simulink model "testboard_UW_GNCDE"  (R2019a)
settings: Solver=FixedStepAuto  StartTime=0.0  StopTime=100  FixedStep=0.05  RelTol=1e-3
values from neighbouring files (symbols this model uses):
  D = zeros(6,3)    [MPCController_test.m]
undefined symbols (not defined in the file or in its folder): Continuous, DiscIntNeverNeededParam, MPCController_test, MPCController_testq, Time
libraries: aerolibutil x23, sharedtransform x5, simulink_extras x4, simulink x4, sharedutil x4, ephemeris x3, sb_quatrans x3, ATV_cowell_plus_tides x2, FO_frame_q x2, FO_ang_vel x2, reference_frame_inv_change x2, sb_qua2con x2
(part 3 of 3)

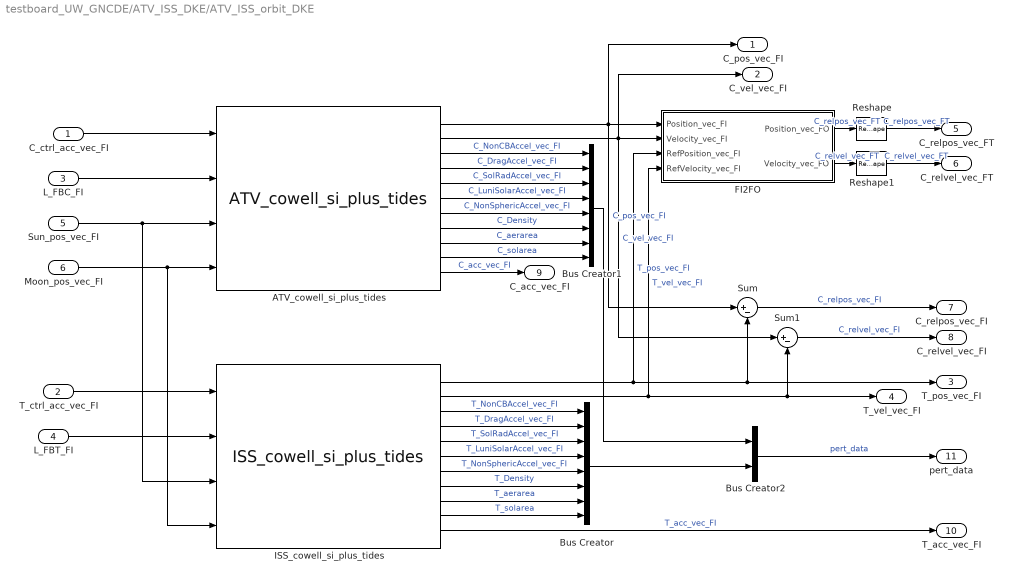
== system testboard_UW_GNCDE/ATV_ISS_DKE/ATV_ISS_orbit_DKE ==
  C_ctrl_acc_vec_FI : Inport
  T_ctrl_acc_vec_FI : Inport  Port=2
  L_FBC_FI : Inport  Port=3
  L_FBT_FI : Inport  Port=4
  Sun_pos_vec_FI : Inport  Port=5
  Moon_pos_vec_FI : Inport  Port=6
  ATV_cowell_si_plus_tides : ATV_cowell_plus_tides/ATV_cowell_si_plus_tides  DiagCtrlNo=6  Ini_option=Specify via Dialog  InitFileName=RVDLEO_test_ATV_cowell_si_plus_tides_init.m  NewFile_Action=Cancel  OldFile_Action=Cancel  InitStatus=on  Ini_Epoch=5479  SC=struct('Ini_Position_vec_FI',[6828447.574;-6.2113;-7.8374],'Ini_Velocity_vec_FI',[3.9161017425529252;4745.7279805152566;5987.6184957602281],'Mass',10,'Cd',2.5,'ReflecCoef',1.3,'stype',3,'aeroa0',0,'solara0',0,'aerob',0,'solarb',0,'XCBdim',0.03,'YCBdim',0.02,'ZCBdim',0.06,'XSAdim',0.03,'YSAdim',0,'ZSAdim',0.06,'SAOrientation',-3,'AeroDragSurface',21,'SolRadSurface',40,'RES_MAG_DIR',1.0000000000000001e-05,'RES_MAG',[1 1 1],'C_COM_FGC',[0 0 0])  AeroDrag_flag=1  SolRad_flag=1  LuniSolar_flag=1  NonSpheric_flag=1  NumZonalTerms=8  NumTessTerms=2  Constants=struct('EarthRadius',6378137,'EarthMu',398600448073446,'SunMu',132712438000000010000,'MoonMu',4902799063000,'SolRadConstant',99060619577789600,'EarthDipoleLong',2.9426251188624395,'EarthDipoleCoelev',1.9120081955597878,'EarthDipole',7943000000000000)
  Bus Creator : BusCreator  Inputs=8
  Bus Creator1 : BusCreator  Inputs=8
  Bus Creator2 : BusCreator  Inputs=2
  FI2FO : Subsystem  AncestorBlock=FI_2_FO/FI2FO
  ISS_cowell_si_plus_tides : ISS_cowell_plus_tides/ISS_cowell_si_plus_tides  DiagCtrlNo=6  Ini_option=Specify via Dialog  InitFileName=RVDLEO_test_ISS_cowell_si_plus_tides_init.m  NewFile_Action=Cancel  OldFile_Action=Cancel  InitStatus=on  Ini_Epoch=5479  SC=struct('Ini_Position_vec_FI',[6828447.574;0;0],'Ini_Velocity_vec_FI',[0;4745.7279805152566;5987.6184957602281],'Mass',10,'Cd',2.5,'ReflecCoef',1.3,'stype',3,'aeroa0',0,'solara0',0,'aerob',0,'solarb',0,'XCBdim',0.03,'YCBdim',0.02,'ZCBdim',0.06,'XSAdim',0.03,'YSAdim',0,'ZSAdim',0.06,'SAOrientation',-3,'AeroDragSurface',0.02,'SolRadSurface',0.06)  AeroDrag_flag=1  SolRad_flag=1  LuniSolar_flag=1  NonSpheric_flag=1  NumZonalTerms=8  NumTessTerms=2  Constants=struct('EarthRadius',6378137,'EarthMu',398600448073446,'SunMu',132712438000000010000,'MoonMu',4902799063000,'SolRadConstant',99060619577789600,'EarthDipoleLong',2.9426251188624395,'EarthDipoleCoelev',1.9120081955597878,'EarthDipole',7943000000000000)
  Reshape : Reshape
  Reshape1 : Reshape
  Sum : Sum  Inputs=|+-  SaturateOnIntegerOverflow=on  InputSameDT=on  OutDataTypeStr=Inherit: Same as first input
  Sum1 : Sum  Inputs=|+-  SaturateOnIntegerOverflow=on  InputSameDT=on  OutDataTypeStr=Inherit: Same as first input
  C_pos_vec_FI : Outport
  C_vel_vec_FI : Outport  Port=2
  T_pos_vec_FI : Outport  Port=3
  T_vel_vec_FI : Outport  Port=4
  C_relpos_vec_FT : Outport  Port=5
  C_relvel_vec_FT : Outport  Port=6
  C_relpos_vec_FI : Outport  Port=7
  C_relvel_vec_FI : Outport  Port=8
  C_acc_vec_FI : Outport  Port=9
  T_acc_vec_FI : Outport  Port=10
  pert_data : Outport  Port=11
  wires:
  Bus Creator/1 -> Bus Creator2/2
  Bus Creator1/1 -> Bus Creator2/1
  ISS_cowell_si_plus_tides/10 -> Bus Creator/8  "T_solarea"
  ISS_cowell_si_plus_tides/9 -> Bus Creator/7  "T_aerarea"
  ISS_cowell_si_plus_tides/8 -> Bus Creator/6  "T_Density"
  ISS_cowell_si_plus_tides/7 -> Bus Creator/5  "T_NonSphericAccel_vec_FI"
  ISS_cowell_si_plus_tides/6 -> Bus Creator/4  "T_LuniSolarAccel_vec_FI"
  ISS_cowell_si_plus_tides/5 -> Bus Creator/3  "T_SolRadAccel_vec_FI"
  ISS_cowell_si_plus_tides/4 -> Bus Creator/2  "T_DragAccel_vec_FI"
  ISS_cowell_si_plus_tides/3 -> Bus Creator/1  "T_NonCBAccel_vec_FI"
  L_FBT_FI/1 -> ISS_cowell_si_plus_tides/2
  T_ctrl_acc_vec_FI/1 -> ISS_cowell_si_plus_tides/1
  Moon_pos_vec_FI/1 -> ATV_cowell_si_plus_tides/4, ISS_cowell_si_plus_tides/4
  Sun_pos_vec_FI/1 -> ATV_cowell_si_plus_tides/3, ISS_cowell_si_plus_tides/3
  L_FBC_FI/1 -> ATV_cowell_si_plus_tides/2
  C_ctrl_acc_vec_FI/1 -> ATV_cowell_si_plus_tides/1
  ATV_cowell_si_plus_tides/10 -> Bus Creator1/8  "C_solarea"
  ATV_cowell_si_plus_tides/8 -> Bus Creator1/6  "C_Density"
  ATV_cowell_si_plus_tides/7 -> Bus Creator1/5  "C_NonSphericAccel_vec_FI"
  ATV_cowell_si_plus_tides/6 -> Bus Creator1/4  "C_LuniSolarAccel_vec_FI"
  ATV_cowell_si_plus_tides/5 -> Bus Creator1/3  "C_SolRadAccel_vec_FI"
  ATV_cowell_si_plus_tides/4 -> Bus Creator1/2  "C_DragAccel_vec_FI"
  ATV_cowell_si_plus_tides/3 -> Bus Creator1/1  "C_NonCBAccel_vec_FI"
  ISS_cowell_si_plus_tides/11 -> T_acc_vec_FI/1  "T_acc_vec_FI"
  ATV_cowell_si_plus_tides/11 -> C_acc_vec_FI/1  "C_acc_vec_FI"
  Bus Creator2/1 -> pert_data/1  "pert_data"
  Sum1/1 -> C_relvel_vec_FI/1  "C_relvel_vec_FI"
  Sum/1 -> C_relpos_vec_FI/1  "C_relpos_vec_FI"
  Reshape1/1 -> C_relvel_vec_FT/1  "C_relvel_vec_FT"
  Reshape/1 -> C_relpos_vec_FT/1  "C_relpos_vec_FT"
  ISS_cowell_si_plus_tides/2 -> T_vel_vec_FI/1, Sum1/2, FI2FO/4(RefVelocity_vec_FI)  "T_vel_vec_FI"
  ISS_cowell_si_plus_tides/1 -> Sum/2, T_pos_vec_FI/1, FI2FO/3(RefPosition_vec_FI)  "T_pos_vec_FI"
  ATV_cowell_si_plus_tides/2 -> C_vel_vec_FI/1, Sum1/1, FI2FO/2(Velocity_vec_FI)  "C_vel_vec_FI"
  ATV_cowell_si_plus_tides/1 -> Sum/1, FI2FO/1(Position_vec_FI), C_pos_vec_FI/1  "C_pos_vec_FI"
  ATV_cowell_si_plus_tides/9 -> Bus Creator1/7  "C_aerarea"
  FI2FO/1(Position_vec_FO) -> Reshape/1  "C_relpos_vec_FT"
  FI2FO/2(Velocity_vec_FO) -> Reshape1/1  "C_relvel_vec_FT"

== system testboard_UW_GNCDE/Dynamic Prototype/Chaser attitude1 ==
  Torque : Inport
  Integrator : Integrator  InitialCondition="[0.2685   -0.1449    0.1277  0.9437]"
  Integrator2 : Integrator  InitialCondition=[2 2 2]*pi/180
  Mux : Mux  Inputs=3
  Mux1 : Mux  Inputs=2
  Td : Constant  Value=ones(3,1)*1e-4
  qdot : MATLABFcn  MATLABFcn=qdot  OutputDimensions=4
  qnorm : MATLAB Function  Commented=on  TreatAsAtomicUnit=on
  wdot1 : MATLABFcn  MATLABFcn=wdot_c  OutputDimensions=3
  q_chaser : Outport
  w_chaser : Outport  Port=2
  wires:
  Integrator2/1 -> Mux1/2, Mux/1, w_chaser/1
  Torque/1 -> Mux/3
  wdot1/1 -> Integrator2/1
  Mux/1 -> wdot1/1
  qdot/1 -> Integrator/1
  Mux1/1 -> qdot/1
  Integrator/1 -> q_chaser/1, Mux1/1
  Td/1 -> Mux/2

== system testboard_UW_GNCDE/Dynamic Prototype/Subsystem1 ==
  q_c : Inport
  q_t : Inport  Port=2
  Quaternion Inverse : aerolibutil/Quaternion Inverse
      settings: SourceProductName=Aerospace Blockset
  Quaternion Multiplication : aerolibutil/Quaternion Multiplication
  q_error : Outport
  wires:
  q_t/1 -> Quaternion Multiplication/1
  q_c/1 -> Quaternion Inverse/1
  Quaternion Inverse/1 -> Quaternion Multiplication/2
  Quaternion Multiplication/1 -> q_error/1

== system testboard_UW_GNCDE/Dynamic Prototype/Target attitude1 ==
  Integrator : Integrator  InitialCondition=[0 0 0 1]
  Integrator2 : Integrator  InitialCondition=[2 2 2]*pi/180*0.01
  MATLAB Function : MATLAB Function  Commented=on  TreatAsAtomicUnit=on
  Mux1 : Mux  Inputs=2
  qdot : MATLABFcn  MATLABFcn=qdot  OutputDimensions=4
  wdot_t : MATLABFcn  MATLABFcn=wdot_t  OutputDimensions=3
  q_target : Outport
  w_target : Outport  Port=2
  wires:
  wdot_t/1 -> Integrator2/1
  Mux1/1 -> qdot/1
  qdot/1 -> Integrator/1
  Integrator/1 -> q_target/1, Mux1/1
  Integrator2/1 -> wdot_t/1, w_target/1, Mux1/2

== system testboard_UW_GNCDE/RVDsensor/coordinate ==
  q_FI_FC : Inport
  q_FI_FT : Inport  Port=2
  Discrete Derivative : simulink/Discrete/Discrete Derivative  gainval=1  ICPrevScaledInput=0.0  OutMin=[]  OutMax=[]  OutDataType=fixdt(1, 16)  OutScaling=2^-10  DoSatur=off
  MATLAB Function1 : MATLAB Function  TreatAsAtomicUnit=on
  Quaternion Multiplication : aerolibutil/Quaternion Multiplication
  Random Number : RandomNumber  Mean=[0;0;0]  Variance=[0.003;0.003;0.003]*0  Seed=[0;0;0]  SampleTime=0.05
  Rotation Angles to Quaternions : sharedtransform/Rotation Angles to Quaternions  rotationOrder=ZYX  aMode=aMode
      settings: SourceProductName=Aerospace Blockset  SourceProductBaseCode=AE
  Unit Delay : UnitDelay  InitialCondition=[0.9515;0.0381;0.1893;0.2393]  SampleTime=-1  HasFrameUpgradeWarning=on
  q_t2c : Subsystem
  RVD_q_FI_FT : Outport
  RVD_w_FT : Outport  Port=2
  wires:
  q_FI_FT/1 -> q_t2c/2(q_t)
  q_FI_FC/1 -> q_t2c/1(q_c)
  Discrete Derivative/1 -> MATLAB Function1/2(qe)
  MATLAB Function1/1(w) -> RVD_w_FT/1
  q_t2c/1(RVD_q_FI_FT) -> Quaternion Multiplication/1
  Unit Delay/1 -> MATLAB Function1/1(u)
  Random Number/1 -> Rotation Angles to Quaternions/1
  Quaternion Multiplication/1 -> Discrete Derivative/1, Unit Delay/1, RVD_q_FI_FT/1
  Rotation Angles to Quaternions/1 -> Quaternion Multiplication/2

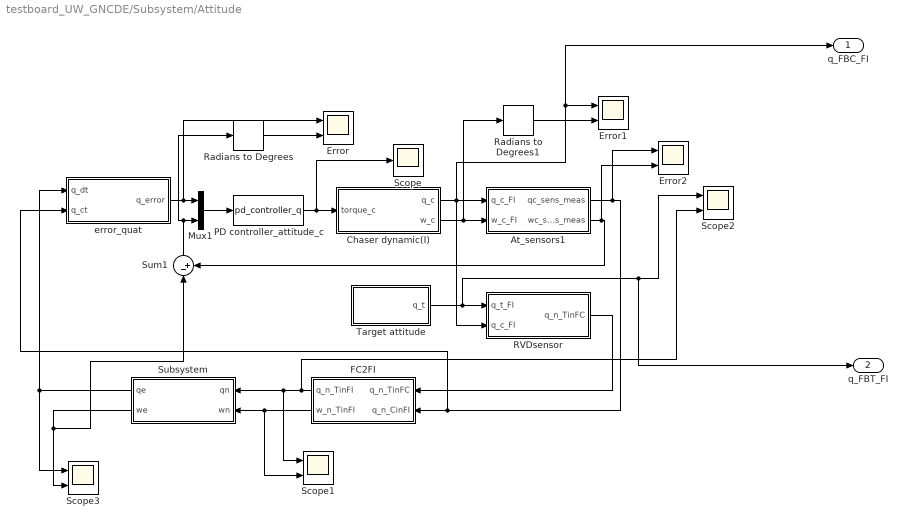
== system testboard_UW_GNCDE/Subsystem/Attitude ==
  At_sensors1 : Subsystem
  Chaser dynamic(I) : Subsystem
  Error : Scope  NumInputPorts=2
  Error1 : Scope  NumInputPorts=2
  Error2 : Scope  NumInputPorts=2
  FC2FI : Subsystem
  Mux1 : Mux  Inputs=2
  PD controller_attitude_c : MATLABFcn  MATLABFcn=pd_controller_q  OutputDimensions=3
  RVDsensor : Subsystem
  Radians to Degrees : simulink_extras/Transformations/Radians to Degrees
  Radians to Degrees1 : simulink_extras/Transformations/Radians to Degrees
  Scope : Scope
  Scope1 : Scope  NumInputPorts=2
  Scope2 : Scope  NumInputPorts=2
  Scope3 : Scope  NumInputPorts=2
  Subsystem : Subsystem
  Sum1 : Sum  Inputs=|-+
  Target attitude : Subsystem
  error_quat : Subsystem
  q_FBC_FI : Outport
  q_FBT_FI : Outport  Port=2
  wires:
  FC2FI/1(q_n_TinFI) -> Scope2/2, Scope1/1, Subsystem/1(qn)
  error_quat/1(q_error) -> Error/1, Mux1/1
  Radians to Degrees1/1 -> Error1/2
  Subsystem/1(qe) -> error_quat/1(q_dt), Scope3/1
  Subsystem/2(we) -> Sum1/1, Scope3/2
  RVDsensor/1(q_n_TinFC) -> FC2FI/1(q_n_TinFC)
  Radians to Degrees/1 -> Error/2
  FC2FI/2(w_n_TinFI) -> Scope1/2, Subsystem/2(wn)
  At_sensors1/2(wc_sens_meas) -> Error2/2, Sum1/2
  Sum1/1 -> Radians to Degrees/1, Mux1/2
  Chaser dynamic(I)/2(w_c) -> Radians to Degrees1/1, At_sensors1/2(w_c_FI)
  Mux1/1 -> PD controller_attitude_c/1
  PD controller_attitude_c/1 -> Scope/1, Chaser dynamic(I)/1(torque_c)
  At_sensors1/1(qc_sens_meas) -> Error2/1, error_quat/2(q_ct), FC2FI/2(q_n_CinFI)
  Chaser dynamic(I)/1(q_c) -> RVDsensor/2(q_c_FI), At_sensors1/1(q_c_FI), q_FBC_FI/1, Error1/1
  Target attitude/1(q_t) -> q_FBT_FI/1, Scope2/1, RVDsensor/1(q_t_FI)

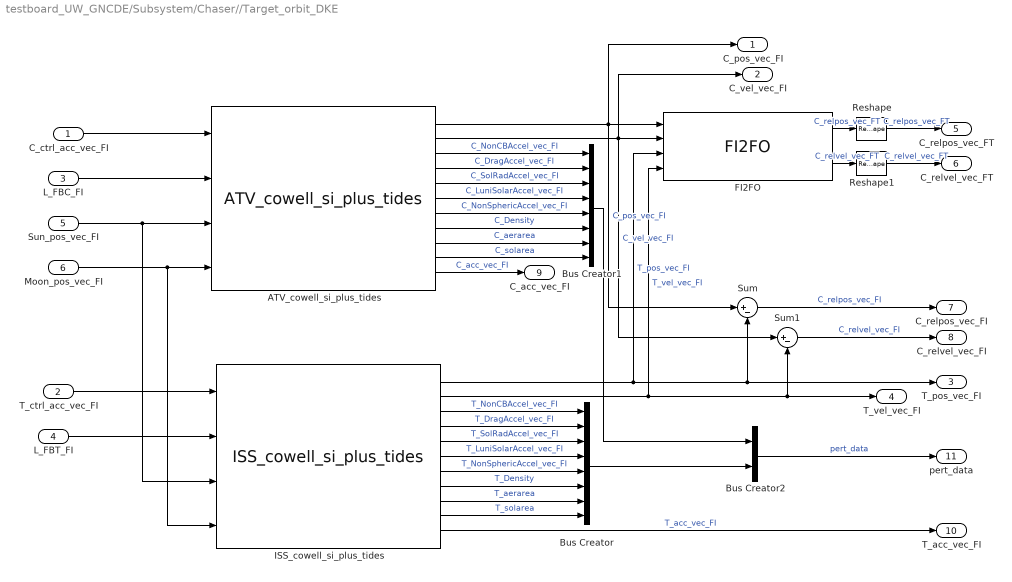
== system testboard_UW_GNCDE/Subsystem/Chaser//Target_orbit_DKE ==
  C_ctrl_acc_vec_FI : Inport
  T_ctrl_acc_vec_FI : Inport  Port=2
  L_FBC_FI : Inport  Port=3
  L_FBT_FI : Inport  Port=4
  Sun_pos_vec_FI : Inport  Port=5
  Moon_pos_vec_FI : Inport  Port=6
  ATV_cowell_si_plus_tides : ATV_cowell_plus_tides/ATV_cowell_si_plus_tides  DiagCtrlNo=6  Ini_option=Specify via Dialog  InitFileName=D:\GNCDE\working_folder\ATV_cowell_si_plus_tides_init.m  NewFile_Action=Cancel  OldFile_Action=Cancel  InitStatus=on  Ini_Epoch=5479  SC=struct('Ini_Position_vec_FI',[6828447.574;-2174.0172420255426;-2742.9270918811635],'Ini_Velocity_vec_FI',[3.9161017425529252;4745.7279805152566;5987.6184957602281],'Mass',10,'Cd',2.5,'ReflecCoef',1.3,'stype',3,'aeroa0',0,'solara0',0,'aerob',0,'solarb',0,'XCBdim',9,'YCBdim',4.5,'ZCBdim',4.5,'XSAdim',0,'YSAdim',5.5,'ZSAdim',5.5,'SAOrientation',-3,'AeroDragSurface',21,'SolRadSurface',40,'RES_MAG_DIR',1.0000000000000001e-05,'RES_MAG',[1 1 1],'C_COM_FGC',[0 0 0])  AeroDrag_flag=1  SolRad_flag=1  LuniSolar_flag=1  NonSpheric_flag=1  NumZonalTerms=8  NumTessTerms=2  Constants=struct('EarthRadius',6378137,'EarthMu',398600448073446,'SunMu',132712438000000010000,'MoonMu',4902799063000,'SolRadConstant',99060619577789600,'EarthDipoleLong',2.9426251188624395,'EarthDipoleCoelev',1.9120081955597878,'EarthDipole',7943000000000000)
  Bus Creator : BusCreator  Inputs=8
  Bus Creator1 : BusCreator  Inputs=8
  Bus Creator2 : BusCreator  Inputs=2
  FI2FO : FI_2_FO/FI2FO  SystemSampleTime=-1
  ISS_cowell_si_plus_tides : ISS_cowell_plus_tides/ISS_cowell_si_plus_tides  DiagCtrlNo=6  Ini_option=Specify via Dialog  InitFileName=D:\GNCDE\working_folder\ISS_cowell_si_plus_tides_init.m  NewFile_Action=Cancel  OldFile_Action=Cancel  InitStatus=on  Ini_Epoch=5479  SC=struct('Ini_Position_vec_FI',[6828447.574;0;0],'Ini_Velocity_vec_FI',[0;4745.7279805152566;5987.6184957602281],'Mass',10,'Cd',2.5,'ReflecCoef',1.3,'stype',3,'aeroa0',0,'solara0',0,'aerob',0,'solarb',0,'XCBdim',54,'YCBdim',65,'ZCBdim',15,'XSAdim',0,'YSAdim',0,'ZSAdim',0,'SAOrientation',-3,'AeroDragSurface',1000,'SolRadSurface',1600)  AeroDrag_flag=1  SolRad_flag=1  LuniSolar_flag=1  NonSpheric_flag=1  NumZonalTerms=8  NumTessTerms=2  Constants=struct('EarthRadius',6378137,'EarthMu',398600448073446,'SunMu',132712438000000010000,'MoonMu',4902799063000,'SolRadConstant',99060619577789600,'EarthDipoleLong',2.9426251188624395,'EarthDipoleCoelev',1.9120081955597878,'EarthDipole',7943000000000000)
  Reshape : Reshape
  Reshape1 : Reshape
  Sum : Sum  Inputs=|+-  SaturateOnIntegerOverflow=on  InputSameDT=on  OutDataTypeStr=Inherit: Same as first input
  Sum1 : Sum  Inputs=|+-  SaturateOnIntegerOverflow=on  InputSameDT=on  OutDataTypeStr=Inherit: Same as first input
  C_pos_vec_FI : Outport
  C_vel_vec_FI : Outport  Port=2
  T_pos_vec_FI : Outport  Port=3
  T_vel_vec_FI : Outport  Port=4
  C_relpos_vec_FT : Outport  Port=5
  C_relvel_vec_FT : Outport  Port=6
  C_relpos_vec_FI : Outport  Port=7
  C_relvel_vec_FI : Outport  Port=8
  C_acc_vec_FI : Outport  Port=9
  T_acc_vec_FI : Outport  Port=10
  pert_data : Outport  Port=11
  wires:
  Bus Creator/1 -> Bus Creator2/2
  Bus Creator1/1 -> Bus Creator2/1
  ISS_cowell_si_plus_tides/10 -> Bus Creator/8  "T_solarea"
  ISS_cowell_si_plus_tides/9 -> Bus Creator/7  "T_aerarea"
  ISS_cowell_si_plus_tides/8 -> Bus Creator/6  "T_Density"
  ISS_cowell_si_plus_tides/7 -> Bus Creator/5  "T_NonSphericAccel_vec_FI"
  ISS_cowell_si_plus_tides/6 -> Bus Creator/4  "T_LuniSolarAccel_vec_FI"
  ISS_cowell_si_plus_tides/5 -> Bus Creator/3  "T_SolRadAccel_vec_FI"
  ISS_cowell_si_plus_tides/4 -> Bus Creator/2  "T_DragAccel_vec_FI"
  ISS_cowell_si_plus_tides/3 -> Bus Creator/1  "T_NonCBAccel_vec_FI"
  L_FBT_FI/1 -> ISS_cowell_si_plus_tides/2
  T_ctrl_acc_vec_FI/1 -> ISS_cowell_si_plus_tides/1
  Moon_pos_vec_FI/1 -> ATV_cowell_si_plus_tides/4, ISS_cowell_si_plus_tides/4
  Sun_pos_vec_FI/1 -> ATV_cowell_si_plus_tides/3, ISS_cowell_si_plus_tides/3
  L_FBC_FI/1 -> ATV_cowell_si_plus_tides/2
  C_ctrl_acc_vec_FI/1 -> ATV_cowell_si_plus_tides/1
  ATV_cowell_si_plus_tides/10 -> Bus Creator1/8  "C_solarea"
  ATV_cowell_si_plus_tides/8 -> Bus Creator1/6  "C_Density"
  ATV_cowell_si_plus_tides/7 -> Bus Creator1/5  "C_NonSphericAccel_vec_FI"
  ATV_cowell_si_plus_tides/6 -> Bus Creator1/4  "C_LuniSolarAccel_vec_FI"
  ATV_cowell_si_plus_tides/5 -> Bus Creator1/3  "C_SolRadAccel_vec_FI"
  ATV_cowell_si_plus_tides/4 -> Bus Creator1/2  "C_DragAccel_vec_FI"
  ATV_cowell_si_plus_tides/3 -> Bus Creator1/1  "C_NonCBAccel_vec_FI"
  ISS_cowell_si_plus_tides/11 -> T_acc_vec_FI/1  "T_acc_vec_FI"
  ATV_cowell_si_plus_tides/11 -> C_acc_vec_FI/1  "C_acc_vec_FI"
  Bus Creator2/1 -> pert_data/1  "pert_data"
  Sum1/1 -> C_relvel_vec_FI/1  "C_relvel_vec_FI"
  Sum/1 -> C_relpos_vec_FI/1  "C_relpos_vec_FI"
  Reshape1/1 -> C_relvel_vec_FT/1  "C_relvel_vec_FT"
  Reshape/1 -> C_relpos_vec_FT/1  "C_relpos_vec_FT"
  ISS_cowell_si_plus_tides/2 -> T_vel_vec_FI/1, Sum1/2, FI2FO/4  "T_vel_vec_FI"
  ISS_cowell_si_plus_tides/1 -> Sum/2, T_pos_vec_FI/1, FI2FO/3  "T_pos_vec_FI"
  ATV_cowell_si_plus_tides/2 -> C_vel_vec_FI/1, Sum1/1, FI2FO/2  "C_vel_vec_FI"
  ATV_cowell_si_plus_tides/1 -> Sum/1, FI2FO/1, C_pos_vec_FI/1  "C_pos_vec_FI"
  ATV_cowell_si_plus_tides/9 -> Bus Creator1/7  "C_aerarea"
  FI2FO/1 -> Reshape/1  "C_relpos_vec_FT"
  FI2FO/2 -> Reshape1/1  "C_relvel_vec_FT"

== system testboard_UW_GNCDE/Subsystem/Ephemeris_postpro ==
  In1 : Inport
  Bus Creator : BusCreator  Inputs=2
  Bus Selector : BusSelector  OutputSignals=Earth_pos_FI,Moon_pos_FI,Sun_pos_FI
  Demux : Demux  Outputs=1
  Sum : Sum  Inputs=-+|
  Sun_pos_vec : Outport
  Moon_pos_vec : Outport  Port=2
  ephemeris_data : Outport  Port=3
  wires:
  Bus Creator/1 -> ephemeris_data/1
  In1/1 -> Bus Selector/1
  Bus Selector/3 -> Sum/2  "<Sun_pos_FI>"
  Bus Selector/2 -> Demux/1  "<Moon_pos_FI>"
  Bus Selector/1 -> Sum/1  "<Earth_pos_FI>"
  Sum/1 -> Bus Creator/2, Sun_pos_vec/1  "Sun_pos_FI"
  Demux/1 -> Bus Creator/1, Moon_pos_vec/1  "Moon_pos_FI"

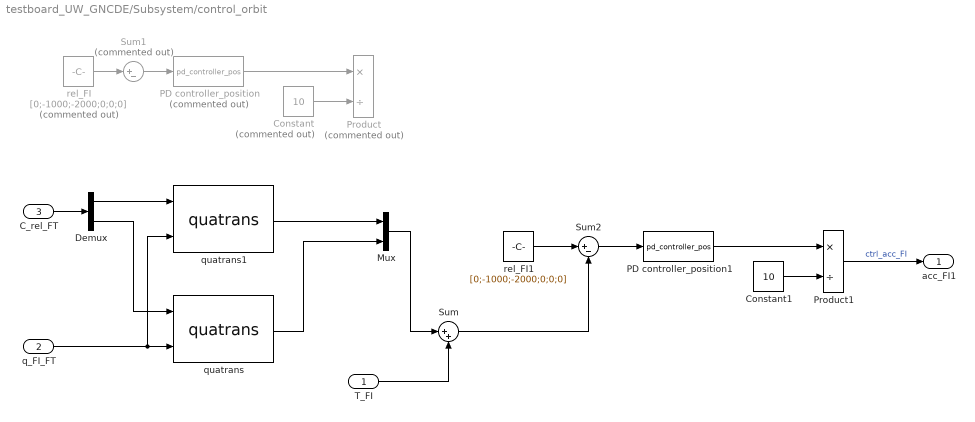
== system testboard_UW_GNCDE/Subsystem/control_orbit ==
  T_FI : Inport
  q_FI_FT : Inport  Port=2
  C_rel_FT : Inport  Port=3
  Constant : Constant  Commented=on  Value=10
  Constant1 : Constant  Value=10
  Demux : Demux  Outputs=2
  Mux : Mux  Inputs=2
  PD controller_position : MATLABFcn  Commented=on  MATLABFcn=pd_controller_pos  OutputDimensions=3
  PD controller_position1 : MATLABFcn  MATLABFcn=pd_controller_pos  OutputDimensions=3
  Product : Product  Commented=on  Inputs=*/  SaturateOnIntegerOverflow=on  RndMeth=Zero  InputSameDT=on  OutDataTypeStr=Inherit: Same as first input
  Product1 : Product  Inputs=*/  SaturateOnIntegerOverflow=on  RndMeth=Zero  InputSameDT=on  OutDataTypeStr=Inherit: Same as first input
  Sum : Sum  Inputs=|++
  Sum1 : Sum  Commented=on  Inputs=|+-
  Sum2 : Sum  Inputs=|+-
  quatrans : sb_quatrans/quatrans
  quatrans1 : sb_quatrans/quatrans
  rel_FI : Constant  Commented=on  Value=[0;-1000;-2000;0;0;0]
  rel_FI1 : Constant  Value=[0;-1000;-2000;0;0;0]
  acc_FI1 : Outport
  wires:
  rel_FI/1 -> Sum1/1
  Sum1/1 -> PD controller_position/1
  PD controller_position/1 -> Product/1
  Constant/1 -> Product/2
  Demux/2 -> quatrans/1
  q_FI_FT/1 -> quatrans1/2, quatrans/2
  quatrans/1 -> Mux/2
  T_FI/1 -> Sum/2
  Sum/1 -> Sum2/2
  Sum2/1 -> PD controller_position1/1
  PD controller_position1/1 -> Product1/1
  Product1/1 -> acc_FI1/1  "ctrl_acc_FI"
  Constant1/1 -> Product1/2
  C_rel_FT/1 -> Demux/1
  Demux/1 -> quatrans1/1
  quatrans1/1 -> Mux/1
  Mux/1 -> Sum/1
  rel_FI1/1 -> Sum2/1

== system testboard_UW_GNCDE/ATV_ISS_DKE/ATV_ISS_orbit_DKE/FI2FO ==
  Position_vec_FI : Inport
  Velocity_vec_FI : Inport  Port=2
  RefPosition_vec_FI : Inport  Port=3
  RefVelocity_vec_FI : Inport  Port=4
  3x3 to 9x1 : Reshape  OutputDimensionality=Customize  OutputDimensions=[9,1]
  FO_frame : FO_frame_q/FO_frame  SystemSampleTime=-1
  RRRAngvel : FO_ang_vel/RRRAngvel  SystemSampleTime=-1
      settings: AttributesFormatString=FO_Angvel
  Reference frame inverse change : reference_frame_inv_change/Reference frame inverse change  SystemSampleTime=-1
      settings: AttributesFormatString=Reference frame inverse change
  qua2con : sb_qua2con/qua2con
  qua2dcm1 : sb_qua2dcm/qua2dcm
  Position_vec_FO : Outport
  Velocity_vec_FO : Outport  Port=2
  wires:
  qua2con/1 -> qua2dcm1/1
  FO_frame/1 -> qua2con/1
  RRRAngvel/1 -> Reference frame inverse change/4
  Reference frame inverse change/1 -> Position_vec_FO/1
  Reference frame inverse change/2 -> Velocity_vec_FO/1
  Velocity_vec_FI/1 -> Reference frame inverse change/2
  Position_vec_FI/1 -> Reference frame inverse change/1
  RefPosition_vec_FI/1 -> RRRAngvel/1, FO_frame/1, Reference frame inverse change/5
  RefVelocity_vec_FI/1 -> RRRAngvel/2, FO_frame/2, Reference frame inverse change/6
  qua2dcm1/1 -> 3x3 to 9x1/1
  3x3 to 9x1/1 -> Reference frame inverse change/3  "L_FO_FI"

== system testboard_UW_GNCDE/RVDsensor/coordinate/q_t2c ==
  note: q_FI_FC
  note: q_FC_FT
  q_c : Inport
  q_t : Inport  Port=2
  Display1 : Display
  Quaternion Conjugate : aerolibutil/Quaternion Conjugate
      settings: SourceProductName=Aerospace Blockset  SourceProductBaseCode=AE
  Quaternion Multiplication : aerolibutil/Quaternion Multiplication
  Quaternion Multiplication1 : aerolibutil/Quaternion Multiplication
  RVD_q_FI_FT : Outport
  wires:
  Quaternion Multiplication/1 -> Quaternion Multiplication1/1
  q_c/1 -> Quaternion Multiplication1/2, Quaternion Conjugate/1
  q_t/1 -> Quaternion Multiplication/1
  Quaternion Conjugate/1 -> Quaternion Multiplication/2
  Quaternion Multiplication1/1 -> Display1/1, RVD_q_FI_FT/1

== system testboard_UW_GNCDE/Subsystem/Attitude/At_sensors1 ==
  q_c_FI : Inport
  w_c_FI : Inport  Port=2
  MATLAB Function : MATLAB Function  TreatAsAtomicUnit=on
  Mux : Mux  Inputs=3
  Quaternion Multiplication : aerolibutil/Quaternion Multiplication
  Random Number : RandomNumber  Variance=(0.003*pi/180)^2  Seed=1  SampleTime=0.1
  Random Number1 : RandomNumber  Variance=(0.003*pi/180)^2  Seed=1  SampleTime=0.1
  Random Number2 : RandomNumber  Variance=(0.007*pi/180)^2  Seed=1  SampleTime=0.1
  Random Number3 : RandomNumber  Mean=[0 0 0]  Variance=[0.01, 0.01, 0.01]*pi/180  Seed=[1 1 1]  SampleTime=0.05
  Sum : Sum  Inputs=|++
  qc_sens_meas : Outport
  wc_sens_meas : Outport  Port=2
  wires:
  Random Number1/1 -> Mux/1
  Random Number/1 -> Mux/2
  Random Number2/1 -> Mux/3
  Mux/1 -> MATLAB Function/1(u)
  MATLAB Function/1(y) -> Quaternion Multiplication/2
  q_c_FI/1 -> Quaternion Multiplication/1
  w_c_FI/1 -> Sum/1
  Random Number3/1 -> Sum/2
  Sum/1 -> wc_sens_meas/1
  Quaternion Multiplication/1 -> qc_sens_meas/1

== system testboard_UW_GNCDE/Subsystem/Attitude/Chaser dynamic(I) ==
  torque_c : Inport
  Discrete-Time Integrator1 : DiscreteIntegrator  InitialCondition=[2 2 2]*pi/180*20  SampleTime=-1  ICPrevOutput=DiscIntNeverNeededParam  ICPrevScaledInput=DiscIntNeverNeededParam
  Discrete-Time Integrator2 : DiscreteIntegrator  InitialCondition="[0.2685   -0.1449    0.1277  0.9437]"  SampleTime=-1  ICPrevOutput=DiscIntNeverNeededParam  ICPrevScaledInput=DiscIntNeverNeededParam
  MATLAB Function : MATLAB Function  TreatAsAtomicUnit=on
  Mux1 : Mux  Inputs=2
  Mux2 : Mux  Inputs=3
  Td : Constant  Value=1*ones(3,1)*1e-4*0
  qdot_c : MATLABFcn  MATLABFcn=qdot_q  OutputDimensions=4
  quat_order : MATLAB Function  TreatAsAtomicUnit=on
  wdot_c : MATLABFcn  MATLABFcn=wdot_c  OutputDimensions=3
  q_c : Outport
  w_c : Outport  Port=2
  wires:
  Discrete-Time Integrator2/1 -> Mux1/1, MATLAB Function/1(u)
  wdot_c/1 -> Discrete-Time Integrator1/1
  Discrete-Time Integrator1/1 -> Mux1/2, w_c/1, Mux2/1
  qdot_c/1 -> Discrete-Time Integrator2/1
  Mux1/1 -> qdot_c/1
  torque_c/1 -> Mux2/3
  Td/1 -> Mux2/2
  Mux2/1 -> wdot_c/1
  MATLAB Function/1(y) -> quat_order/1(u)
  quat_order/1(y) -> q_c/1

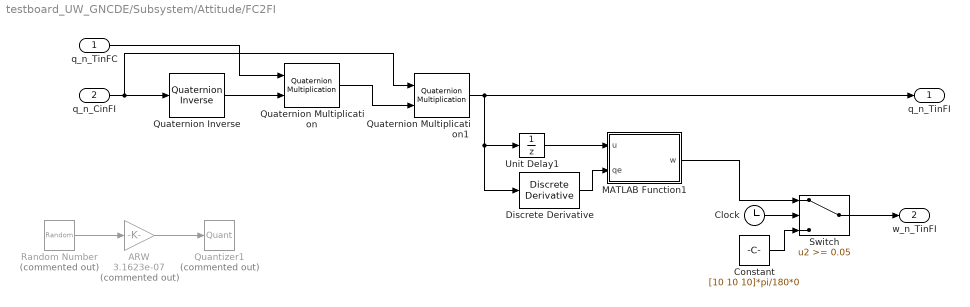
== system testboard_UW_GNCDE/Subsystem/Attitude/FC2FI ==
  q_n_TinFC : Inport
  q_n_CinFI : Inport  Port=2
  ARW : Gain  Commented=on  Gain=3.1623e-07
  Clock : Clock
  Constant : Constant  Value=[10 10 10]*pi/180*0
  Discrete Derivative : simulink/Discrete/Discrete Derivative  gainval=1.0  ICPrevScaledInput="[0.2685   -0.1449    0.1277 0.9437]"  OutMin=[]  OutMax=[]  OutDataType=fixdt(1, 16)  OutScaling=2^-10  DoSatur=off
  MATLAB Function1 : MATLAB Function  TreatAsAtomicUnit=on
  Quantizer1 : Quantizer  Commented=on  QuantizationInterval=1.0000e-08
  Quaternion Inverse : aerolibutil/Quaternion Inverse
      settings: SourceProductName=Aerospace Blockset
  Quaternion Multiplication : aerolibutil/Quaternion Multiplication
  Quaternion Multiplication1 : aerolibutil/Quaternion Multiplication
  Random Number : RandomNumber  Commented=on  Mean=[0 0 0]  Variance=[1 1 1]  Seed=[77 88 99]  SampleTime=0.05
  Switch : Switch  Threshold=0.05
  Unit Delay1 : UnitDelay  InitialCondition=[1;0;0;0]  SampleTime=0.05  HasFrameUpgradeWarning=on
  q_n_TinFI : Outport
  w_n_TinFI : Outport  Port=2
  wires:
  q_n_CinFI/1 -> Quaternion Multiplication1/1, Quaternion Inverse/1
  Quaternion Inverse/1 -> Quaternion Multiplication/2
  q_n_TinFC/1 -> Quaternion Multiplication/1
  Quaternion Multiplication/1 -> Quaternion Multiplication1/2
  Unit Delay1/1 -> MATLAB Function1/1(u)
  Discrete Derivative/1 -> MATLAB Function1/2(qe)
  MATLAB Function1/1(w) -> Switch/1
  Clock/1 -> Switch/2
  Constant/1 -> Switch/3
  Switch/1 -> w_n_TinFI/1
  Quaternion Multiplication1/1 -> q_n_TinFI/1, Discrete Derivative/1, Unit Delay1/1
  ARW/1 -> Quantizer1/1
  Random Number/1 -> ARW/1

== system testboard_UW_GNCDE/Subsystem/Attitude/RVDsensor ==
  q_t_FI : Inport
  q_c_FI : Inport  Port=2
  At_sensors : Subsystem
  q_FT2FC : Subsystem
  q_n_TinFC : Outport
  wires:
  q_t_FI/1 -> q_FT2FC/2(q_t)
  q_c_FI/1 -> q_FT2FC/1(q_c)
  At_sensors/1(sens_meas) -> q_n_TinFC/1
  q_FT2FC/1(q_TinFC) -> At_sensors/1(state)

== system testboard_UW_GNCDE/Subsystem/Attitude/Subsystem ==
  qn : Inport
  wn : Inport  Port=2
  Clock : Clock
  Constant : Constant  Value=[10 10 10]*pi/180*0
  Discrete Derivative : simulink/Discrete/Discrete Derivative  gainval=1.0  ICPrevScaledInput="[0.2685   -0.1449    0.1277 0.9437]"  OutMin=[]  OutMax=[]  OutDataType=fixdt(1, 16)  OutScaling=2^-10  DoSatur=off
  MATLAB Function : MATLAB Function  TreatAsAtomicUnit=on
  MATLAB Function1 : MATLAB Function  TreatAsAtomicUnit=on
  Switch : Switch  Threshold=0.05
  Terminator : Terminator
  Terminator1 : Terminator
  Unit Delay1 : UnitDelay  InitialCondition=[1;0;0;0]  SampleTime=0.05  HasFrameUpgradeWarning=on
  qe : Outport
  we : Outport  Port=2
  wires:
  wn/1 -> MATLAB Function/1(wn)
  qn/1 -> MATLAB Function/2(qn)
  MATLAB Function/3(Kn) -> Terminator/1
  MATLAB Function/2(Pn) -> Terminator1/1
  Constant/1 -> Switch/3
  Discrete Derivative/1 -> MATLAB Function1/2(qe)
  MATLAB Function/1(qe) -> Unit Delay1/1, Discrete Derivative/1, qe/1
  Unit Delay1/1 -> MATLAB Function1/1(u)
  Switch/1 -> we/1
  Clock/1 -> Switch/2
  MATLAB Function1/1(w) -> Switch/1

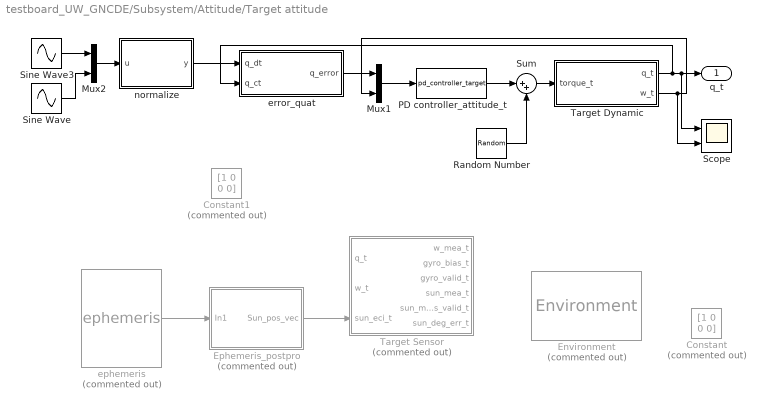
== system testboard_UW_GNCDE/Subsystem/Attitude/Target attitude ==
  Constant : Constant  Commented=on  Value=[1 0 0 0]
  Constant1 : Constant  Commented=on  Value=[1 0 0 0]
  Environment : environment_lib/Environment  Commented=on  SystemSampleTime=-1
  Ephemeris_postpro : Subsystem  Commented=on
  Mux1 : Mux  Inputs=2
  Mux2 : Mux  Inputs=2
  PD controller_attitude_t : MATLABFcn  MATLABFcn=pd_controller_target  OutputDimensions=3
  Random Number : RandomNumber  Mean=[0 0 0]  Variance=[1 1 1]*pi/180*0.0001  Seed=[0 0 0]  SampleTime=0.05
  Scope : Scope  NumInputPorts=2
  Sine Wave : Sin  Amplitude=[1 1 1]  Frequency=[0.01 0.01 0.01]*pi/180  SampleTime=0
  Sine Wave3 : Sin  Frequency=0.01*pi/180  Phase=pi/2  SampleTime=0
  Sum : Sum  Inputs=|++
  Target Dynamic : Subsystem
  Target Sensor : Subsystem  Commented=on
  ephemeris : ephemeris/ephemeris  Commented=on  DiagCtrlNo=6  Ini_option=Specify via Dialog  InitFileName=D:\GNCDE\working_folder\ephemeris_init.m  NewFile_Action=Cancel  OldFile_Action=Cancel  InitStatus=off  Ini_Epoch=0  Enable_Body=[0 0 1 0 0 0 0 0 0 1 1 0 0]  chbycf=struct('EAR',[5109.14071937975 5115.02729345383 10 -21159536960.3208 -7616228246.62673 14130388.7851396 918478.623258763 4006.48713181974 -477.827985971137 -82.624370745598 -0.189251355812849 1.28757540542271 0.0955724834745023 -0.0152204285311983 133152151856.35 -1030925778.19867 -90460120.6721068 78522.2611073916 10706.7288670719 601.288630786409 -22.070788671657 -9.95932429009475 -0.406667183944299 0.136888722970201 0.0170747736826146 57708317032.9772 -447235400.43436 -39188189.7036111 40351.662341568 4443.43282472309 185.251889578774 -12.167621395698 -3.48646683320875 -0.0724173818042665 0.0529313616532479 0.00513332732835961],'MOO',[5112.11065221135 5116.20324480394 10 34650173.993104 186514002.435041 -2495389.26759137 -2174583.68238657 4930.02817645175 12999.0721003394 120.667942375399 -92.5415797256388 -2.14437005881584 0.793634635239226 0.0295435598949569 -313601656.624057 18264721.8031473 22354714.6101463 -124743.704004404 -159772.889741809 -692.804912624185 997.735939260278 17.8198848774754 -7.99248030690066 -0.25294541069076 0.0716620130504439 -108071413.445559 16469962.5763651 7672023.68224794 -161330.902436691 -55425.3288019514 462.342458298577 354.592641593109 1.21305976257097 -2.90631639139957 -0.0453904819226325 0.0266212793197802],'SUN',[5112.01145973333 5114.62229306667 10 147014971.405969 1184271.71104419 -218.919763945895 -0.798352834961094 0.000864658889320531 -1.37580451992723e-05 0 -2.33669146422292e-05 -2.64424988568438e-05 1.92480528795026e-05 2.64233279157347e-05 -307317354.002752 426771.396314319 677.643512396405 -0.135250863530393 -0.00223429398300006 -2.68271044630026e-06 0 -8.38562534430828e-06 -9.55861999364935e-06 6.90255426577262e-06 9.70397461955064e-06 -148398632.203105 155130.899246664 297.438278583177 -0.0362566872851819 -0.00100748145753106 -7.97485362452454e-07 0 -3.04885599201112e-06 -3.46109125688042e-06 2.50296515024027e-06 3.52933846085304e-06;5114.62229306667 5117.2331264 10 149381733.33318 1182482.31702465 -228.395762813599 -0.779967211154815 0 -1.47874999702568e-05 -0.00127166231016246 -2.32635695876312e-05 -2.63511861481436e-05 1.9161193425111e-05 0.000662121720523023 -306458395.616485 432185.468791277 675.81529681803 -0.168583804133088 0 4.2800990604841e-06 0.00196801761717869 -8.42282466766873e-06 -9.68372849448267e-06 6.93061447362379e-06 -0.00097420546790237 -148085992.46425 157508.400514139 296.910058624337 -0.0514142652254682 0 2.83284440005886e-06 0.000896707875385124 -3.05485575406555e-06 -3.53152203162797e-06 2.51591401863033e-06 -0.000444752606548563],'MER',[0 0 0 0 0 0 0 0 0 0 0 0 0 0 0 0 0 0 0 0 0 0 0 0 0 0 0 0 0 0 0 0 0 0 0 0],'VEN',[0 0 0 0 0 0 0 0 0 0 0 0 0 0 0 0 0 0 0 0 0 0 0 0 0 0 0 0 0 0 0 0 0 0 0 0],'MAR',[0 0 0 0 0 0 0 0 0 0 0 0 0 0 0 0 0 0 0 0 0 0 0 0 0 0 0 0 0 0 0 0 0 0 0 0],'JUP',[0 0 0 0 0 0 0 0 0 0 0 0 0 0 0 0 0 0 0 0 0 0 0 0 0 0 0 0 0 0 0 0 0 0 0 0],'SAT',[0 0 0 0 0 0 0 0 0 0 0 0 0 0 0 0 0 0 0 0 0 0 0 0 0 0 0 0 0 0 0 0 0 0 0 0],'URA',[0 0 0 0 0 0 0 0 0 0 0 0 0 0 0 0 0 0 0 0 0 0 0 0 0 0 0 0 0 0 0 0 0 0 0 0],'NEP',[0 0 0 0 0 0 0 0 0 0 0 0 0 0 0 0 0 0 0 0 0 0 0 0 0 0 0 0 0 0 0 0 0 0 0 0],'PLU',[0 0 0 0 0 0 0 0 0 0 0 0 0 0 0 0 0 0 0 0 0 0 0 0 0 0 0 0 0 0 0 0 0 0 0 0],'PHO',[0 0 0 0 0 0 0 0 0 0 0 0 0 0 0 0 0 0 0 0 0 0 0 0 0 0 0 0 0 0 0 0 0 0 0 0],'DEI',[0 0 0 0 0 0 0 0 0 0 0 0 0 0 0 0 0 0 0 0 0 0 0 0 0 0 0 0 0 0 0 0 0 0 0 0])
  error_quat : Subsystem
  normalize : MATLAB Function  TreatAsAtomicUnit=on
  q_t : Outport
  wires:
  ephemeris/1 -> Ephemeris_postpro/1(In1)
  Ephemeris_postpro/1(Sun_pos_vec) -> Target Sensor/3(sun_eci_t)
  Target Dynamic/1(q_t) -> error_quat/2(q_ct), Scope/1, q_t/1
  Target Dynamic/2(w_t) -> Scope/2, Mux1/2
  Sum/1 -> Target Dynamic/1(torque_t)
  Mux1/1 -> PD controller_attitude_t/1
  normalize/1(y) -> error_quat/1(q_dt)
  PD controller_attitude_t/1 -> Sum/1
  error_quat/1(q_error) -> Mux1/1
  Random Number/1 -> Sum/2
  Sine Wave3/1 -> Mux2/1
  Mux2/1 -> normalize/1(u)
  Sine Wave/1 -> Mux2/2

== system testboard_UW_GNCDE/Subsystem/Attitude/error_quat ==
  q_dt : Inport
  q_ct : Inport  Port=2
  Quaternion Inverse : aerolibutil/Quaternion Inverse
      settings: SourceProductName=Aerospace Blockset
  Quaternion Multiplication : aerolibutil/Quaternion Multiplication
  q_error : Outport
  wires:
  q_dt/1 -> Quaternion Inverse/1
  Quaternion Multiplication/1 -> q_error/1
  q_ct/1 -> Quaternion Multiplication/2
  Quaternion Inverse/1 -> Quaternion Multiplication/1

== system testboard_UW_GNCDE/Subsystem/Attitude/RVDsensor/At_sensors ==
  state : Inport
  MATLAB Function : MATLAB Function  Commented=on  TreatAsAtomicUnit=on
  Quaternion Multiplication : aerolibutil/Quaternion Multiplication
  Random Number1 : RandomNumber  Mean=[0 0 0]  Variance=[0.003^2 0.003^2 0.007^2]*pi/180  Seed=[77 88 99]  SampleTime=0.05
  Rotation Angles to Quaternions : sharedtransform/Rotation Angles to Quaternions  rotationOrder=ZYX  aMode=aMode
      settings: SourceProductName=Aerospace Blockset  SourceProductBaseCode=AE
  sens_meas : Outport
  wires:
  Rotation Angles to Quaternions/1 -> Quaternion Multiplication/2
  state/1 -> Quaternion Multiplication/1
  Quaternion Multiplication/1 -> sens_meas/1
  Random Number1/1 -> Rotation Angles to Quaternions/1

== system testboard_UW_GNCDE/Subsystem/Attitude/RVDsensor/q_FT2FC ==
  q_c : Inport
  q_t : Inport  Port=2
  Quaternion Inverse : aerolibutil/Quaternion Inverse
      settings: SourceProductName=Aerospace Blockset
  Quaternion Multiplication : aerolibutil/Quaternion Multiplication
  Quaternion Multiplication1 : aerolibutil/Quaternion Multiplication
  q_TinFC : Outport
  wires:
  q_c/1 -> Quaternion Inverse/1, Quaternion Multiplication/2
  q_t/1 -> Quaternion Multiplication/1
  Quaternion Multiplication1/1 -> q_TinFC/1
  Quaternion Inverse/1 -> Quaternion Multiplication1/1
  Quaternion Multiplication/1 -> Quaternion Multiplication1/2

== system testboard_UW_GNCDE/Subsystem/Attitude/Target attitude/Ephemeris_postpro ==
  In1 : Inport
  Bus Selector : BusSelector  OutputSignals=Earth_pos_FI,Sun_pos_FI
  Sum : Sum  Inputs=-+|
  Sun_pos_vec : Outport
  wires:
  In1/1 -> Bus Selector/1
  Bus Selector/2 -> Sum/2  "<Sun_pos_FI>"
  Bus Selector/1 -> Sum/1  "<Earth_pos_FI>"
  Sum/1 -> Sun_pos_vec/1  "Sun_pos_FI"

== system testboard_UW_GNCDE/Subsystem/Attitude/Target attitude/Target Dynamic ==
  torque_t : Inport
  Discrete-Time Integrator : DiscreteIntegrator  InitialCondition=[10 10 10]*pi/180*0  SampleTime=-1  ICPrevOutput=DiscIntNeverNeededParam  ICPrevScaledInput=DiscIntNeverNeededParam
  Discrete-Time Integrator1 : DiscreteIntegrator  InitialCondition=[0.2685 -0.1449 0.1277 0.9437]  SampleTime=-1  ICPrevOutput=DiscIntNeverNeededParam  ICPrevScaledInput=DiscIntNeverNeededParam
  MATLAB Function : MATLAB Function  TreatAsAtomicUnit=on
  Mux1 : Mux  Inputs=2
  Mux2 : Mux  Inputs=3
  Td : Constant  Value=1*ones(3,1)*1e-4*0
  qdot_t : MATLABFcn  MATLABFcn=qdot_q  OutputDimensions=4
  quat_order : MATLAB Function  TreatAsAtomicUnit=on
  wdot_t : MATLABFcn  MATLABFcn=wdot_c  OutputDimensions=3
  q_t : Outport
  w_t : Outport  Port=2
  wires:
  Discrete-Time Integrator1/1 -> MATLAB Function/1(u), Mux1/1
  wdot_t/1 -> Discrete-Time Integrator/1
  Discrete-Time Integrator/1 -> Mux1/2, w_t/1, Mux2/1
  qdot_t/1 -> Discrete-Time Integrator1/1
  Mux1/1 -> qdot_t/1
  torque_t/1 -> Mux2/3
  Td/1 -> Mux2/2
  Mux2/1 -> wdot_t/1
  MATLAB Function/1(y) -> quat_order/1(u)
  quat_order/1(y) -> q_t/1

== system testboard_UW_GNCDE/Subsystem/Attitude/Target attitude/Target Sensor ==
  q_t : Inport
  w_t : Inport  Port=2
  sun_eci_t : Inport  Port=3
  SunSensor : SunSensor/SunSensor  DiagCtrlNo=6  Ini_option=Specify via Dialog  InitFileName=D:\GNCDE\working_folder\SunSensor_init.m  NewFile_Action=Cancel  OldFile_Action=Cancel  InitStatus=off  SC_EA_321_SBF_GFF=[0 0 0]  SAS_alpha_beta_sigma_SRF=[3.046e-06 3.046e-06]  SAS_alpha_beta_noise_seed=[0 1000]  SAS_alpha_beta_bias=[0 0]  SAS_EA_321_ESRF_SRF=[0 0 0]  SAS_EA_321_SRF_GFF=[0 0 0]  SAS_alpha_beta_limit=[3.14159265358979 3.14159265358979]  SAS_sample_time=0.1  SAS_earth_flag=0  SAS_FOV=3.14159265358979  SC_EA_321_RBF_GFF=[0 0 0]
  gyro_sim_lib : gyroscope_lib/gyro_sim_lib  SystemSampleTime=-1
  magnetometer_sim_lib : magnetometer_lib/magnetometer_sim_lib  Commented=on  SystemSampleTime=-1
  sun_sensor_lib : sun_sensor_lib/sun_sensor_lib   SystemSampleTime=-1
  w_mea_t : Outport
  gyro_bias_t : Outport  Port=2
  gyro_valid_t : Outport  Port=3
  sun_mea_t : Outport  Port=4
  sun_meas_valid_t : Outport  Port=5
  sun_deg_err_t : Outport  Port=6
  wires:
  gyro_sim_lib/1 -> w_mea_t/1
  w_t/1 -> gyro_sim_lib/1
  q_t/1 -> sun_sensor_lib/2
  sun_sensor_lib/1 -> sun_mea_t/1
  sun_sensor_lib/2 -> sun_meas_valid_t/1
  sun_sensor_lib/3 -> sun_deg_err_t/1
  gyro_sim_lib/2 -> gyro_bias_t/1
  gyro_sim_lib/3 -> gyro_valid_t/1
  sun_eci_t/1 -> sun_sensor_lib/1

== system testboard_UW_GNCDE/Subsystem/Attitude/Target attitude/error_quat ==
  q_dt : Inport
  q_ct : Inport  Port=2
  Quaternion Inverse : aerolibutil/Quaternion Inverse
      settings: SourceProductName=Aerospace Blockset
  Quaternion Multiplication : aerolibutil/Quaternion Multiplication
  q_error : Outport
  wires:
  q_dt/1 -> Quaternion Inverse/1
  Quaternion Multiplication/1 -> q_error/1
  q_ct/1 -> Quaternion Multiplication/2
  Quaternion Inverse/1 -> Quaternion Multiplication/1

== matlab function testboard_UW_GNCDE/Subsystem/Attitude/RVDsensor/At_sensors/MATLAB Function ==
  data: u input; y output
function y = fcn(u)

eul = [u(1) u(2) u(3)];
y = eul2quat(eul)

== matlab function testboard_UW_GNCDE/Kalman Filter/Kalman Filter ==
  settings: updateMethod=DISCRETE
  data: wn input; qe output; qn input
function qe  = KalF(wn,qn)

%qn = [scalar; vector];
persistent x P

qn = [qn(2); qn(3); qn(4); qn(1)];

if isempty(x)
    x = [0 0 0 1]';
    P = 1*eye(4);
end

dt = 0.05;
A = eye(4)+dt*1/2*[0 wn(3) -wn(2) wn(1);
    -wn(3) 0 wn(1) wn(2);
    wn(2) -wn(1) 0 wn(3);
    -wn(1) -wn(2) -wn(3) 0];
H = eye(4); 
Q = (0.5^2)*eye(4);
R = eye(4);%zeros(4);

xp = A*x;
Pp = A*P*A' + Q;

K=Pp*H'*inv(H*Pp*H'+R);

x=xp+K*(qn-H*xp);
P=Pp-K*H*Pp;

x = [x(4); x(1); x(2); x(3)];
qe=x;

% q=15.25; r=0.0003;
% Q = (q*pi/180)^2*eye(4);  %300 arcsec
%Q = q^2*eye(4);
% dH = [0.5 0 0;
%     0 0.5 0;
%     0 0 0.5;
%     0 0 0];
% Ry = [(r*pi/180)^2 0 0;      %60, 60, 300 arcsec / 0.02, 0.02, 0.1 deg 1초 = 0.000277778도
%       0 (r*pi/180)^2 0;
%       0 0 (r*5*pi/180)^2];
% Ry = [r^2 0 0;      %60, 60, 300 arcsec / 0.02, 0.02, 0.1 deg 1초 = 0.000277778도
%       0 r^2 0;
%       0 0 r^2];
% Rq = dH*Ry*dH';
% Rq = eye(4);
% Qq = [qn(4) qn(3) -qn(2) qn(1);
%     -qn(3) qn(4) qn(1) qn(2);
%     qn(2) -qn(1) qn(4) qn(3);
%     -qn(1) -qn(2) -qn(3) qn(4)];
% R = Qq*Rq*Qq';
% qH = error_quaternion(qn,H*xp);
%kq = K*qH; %(qn-H*xp);
%x=qmult(xp,kq);

== matlab function testboard_UW_GNCDE/RVDsensor/coordinate/MATLAB Function1 ==
  data: u input; w output; qe input
function w = fcn(u,qe)

q = [u(2) u(3) u(4) u(1)];
Q = [q(4) -q(3) q(2) q(1);
    q(3) q(4) -q(1) q(2);
    -q(2) q(1) q(4) q(3);
    -q(1) -q(2) -q(3) q(4)];
qe = [qe(2) qe(3) qe(4) qe(1)]';

W = 2*inv(Q)*qe;
w = [W(1) W(2) W(3)]';

== matlab function testboard_UW_GNCDE/Subsystem/Attitude/Chaser dynamic(I)/MATLAB Function ==
  data: u input; y output
function y = fcn(u)
%#codegen

y = u/norm(u);

== matlab function testboard_UW_GNCDE/Subsystem/Attitude/Subsystem/MATLAB Function ==
  settings: updateMethod=DISCRETE
  data: wn input; qe output; qn input; Pn output; Kn output
function [qe,Pn,Kn] = KF(wn,qn)

persistent x P

qn = [qn(2) qn(3) qn(4) qn(1)]';

if isempty(x)
    x = [0 0 0 1]';
    P = 1*eye(4);
end

dt = 0.05;

A = eye(4)+dt*1/2*[0 wn(3) -wn(2) wn(1);
    -wn(3) 0 wn(1) wn(2);
    wn(2) -wn(1) 0 wn(3);
    -wn(1) -wn(2) -wn(3) 0];
H = eye(4);
q=0.25; %r=1.97;
Q = (q*pi/180)^2*eye(4);  %300 arcsec
dH = [0.5 0 0;
    0 0.5 0;
    0 0 0.5;
    0 0 0];
Ry = [(0.1*pi/180)^2 0 0;      %60, 60, 300 arcsec / 0.02, 0.02, 0.1 deg 1초 = 0.000277778도
      0 (0.1*pi/180)^2 0;
      0 0 (0.1*pi/180)^2];
Rq = dH*Ry*dH';
Qq = [qn(4) qn(3) -qn(2) qn(1);
    -qn(3) qn(4) qn(1) qn(2);
    qn(2) -qn(1) qn(4) qn(3);
    -qn(1) -qn(2) -qn(3) qn(4)];
R = Qq*Rq*Qq';

xp = A*x;
Pp = A*P*A' + Q;

K=Pp*H'*inv(H*Pp*H'+R);
x=xp+K*(qn-H*xp);
P=Pp-K*H*Pp;

qe=x;
qe=[qe(4) qe(1) qe(2) qe(3)]';
Pn=norm(P);
Kn=norm(K);

== matlab function testboard_UW_GNCDE/Subsystem/Attitude/Chaser dynamic(I)/quat_order ==
  data: u input; y output
function y = fcn(u)

y = [u(4) u(1) u(2) u(3)];

== matlab function testboard_UW_GNCDE/Dynamic Prototype/Chaser attitude1/qnorm ==
  data: u input; y output
function y = fcn(u)
%#codegen

y = u/norm(u);

== matlab function testboard_UW_GNCDE/Dynamic Prototype/MATLAB Function1 ==
  data: DCM_toT input; y output; DCM_toC input; u input
function y = DCM_T_to_C(DCM_toT, DCM_toC, u)

y = DCM_toC*DCM_toT'*u;

== matlab function testboard_UW_GNCDE/Dynamic Prototype/Target attitude1/MATLAB Function ==
  data: u input; y output
function y = fcn(u)
%#codegen

y = u/norm(u);

== matlab function testboard_UW_GNCDE/Dynamic Prototype/quat1 ==
  data: u input; y output
function y = fcn(u)

y = [u(4) u(1) u(2) u(3)];

== matlab function testboard_UW_GNCDE/Dynamic Prototype/quat ==
  data: u input; y output
function y = fcn(u)

y = [u(4) u(1) u(2) u(3)];

== matlab function testboard_UW_GNCDE/Dynamic Prototype/dcm_toT ==
  data: u input; y output
function y = fcn(u)

y = quat2dcm2(u);

== matlab function testboard_UW_GNCDE/Dynamic Prototype/dcm_toC ==
  data: u input; y output
function y = fcn(u)

y = quat2dcm2(u);

== matlab function testboard_UW_GNCDE/MATLAB Function ==
  data: wn input; A output
function A = fcn(wn)
dt = 0.05;


A = eye(4)+dt*1/2*[0 wn(3) -wn(2) wn(1);
    -wn(3) 0 wn(1) wn(2);
    wn(2) -wn(1) 0 wn(3);
    -wn(1) -wn(2) -wn(3) 0];

== matlab function testboard_UW_GNCDE/Subsystem1/MATLAB Function4 ==
  data: qn input; y output
function y = fcn(qn)

y = [qn(2); qn(3); qn(4); qn(1)];

== matlab function testboard_UW_GNCDE/Subsystem/Attitude/Subsystem/MATLAB Function1 ==
  data: u input; w output; qe input
function w = fcn(u,qe)

if isempty(qe)
    qe = [1 0 0 0];
    u = [1 0 0 0];
end

q = [u(2) u(3) u(4) u(1)];
Q = [q(4) -q(3) q(2) q(1);
    q(3) q(4) -q(1) q(2);
    -q(2) q(1) q(4) q(3);
    -q(1) -q(2) -q(3) q(4)];
qe = [qe(2) qe(3) qe(4) qe(1)]';

W = 2*inv(Q)*qe;
w = [W(1) W(2) W(3)];

== matlab function testboard_UW_GNCDE/Subsystem2/MATLAB Function4 ==
  data: qn input; y output
function y = fcn(qn)

y = [qn(2); qn(3); qn(4); qn(1)];

== matlab function testboard_UW_GNCDE/MATLAB Function3 ==
  data: y input; qe output
function qe = fcn(y)

qe = [y(4); y(1); y(2); y(3)];

== matlab function testboard_UW_GNCDE/Subsystem/Attitude/At_sensors1/MATLAB Function ==
  data: u input; y output
function y = fcn(u)

eul = [u(1) u(2) u(3)];
y = eul2quat(eul)

== matlab function testboard_UW_GNCDE/Subsystem/Attitude/Target attitude/Target Dynamic/MATLAB Function ==
  data: u input; y output
function y = fcn(u)
%#codegen

y = u/norm(u);

== matlab function testboard_UW_GNCDE/Subsystem/Attitude/Target attitude/Target Dynamic/quat_order ==
  data: u input; y output
function y = fcn(u)

y = [u(4) u(1) u(2) u(3)];

== matlab function testboard_UW_GNCDE/Subsystem/Attitude/Target attitude/normalize ==
  data: u input; y output
function y = fcn(u)
%#codegen

y = u/norm(u);

== matlab function testboard_UW_GNCDE/Subsystem/Attitude/FC2FI/MATLAB Function1 ==
  data: u input; w output; qe input
function w = fcn(u,qe)

if isempty(qe)
    qe = [1 0 0 0];
    u = [1 0 0 0];
end

q = [u(2) u(3) u(4) u(1)];
Q = [q(4) -q(3) q(2) q(1);
    q(3) q(4) -q(1) q(2);
    -q(2) q(1) q(4) q(3);
    -q(1) -q(2) -q(3) q(4)];
qe = [qe(2) qe(3) qe(4) qe(1)]';

W = 2*inv(Q)*qe;
w = [W(1) W(2) W(3)];
